simulink model "TF_TrajectoireFollowing_Segment"  (R2021b)
settings: Solver=FixedStepAuto  StartTime=0.0  StopTime=100  FixedStep=sampleTime  RelTol=1e-3  EnableMultiTasking=on
values from neighbouring files (symbols this model uses):
  k_d_x = 1.5    [startSimulation.m]
  k_d_y = 1.5    [startSimulation.m]
  k_d_yaw = 1    [startSimulation.m]
  k_d_z = 0.5    [startSimulation.m]
  k_i_x = 0.01    [startSimulation.m]
  k_i_y = 0.01    [startSimulation.m]
  k_i_yaw = 0.01    [startSimulation.m]
  k_i_z = 0.01    [startSimulation.m]
  k_p_x = 1.2    [startSimulation.m]
  k_p_y = 1.5    [startSimulation.m]
  k_p_yaw = 2    [startSimulation.m]
  k_p_z = 2    [startSimulation.m]
  saturation_psi = 2    [startSimulation.m]
  saturation_x = 2    [startSimulation.m]
  saturation_y = 2    [startSimulation.m]
  saturation_z = 2    [startSimulation.m]
libraries: simulink x28, aerolibanimutils x1
settings Model: Creator=exbot  LastModifiedBy=Lenovo
settings SolverCC: AlgebraicLoopSolver=TrustRegion
settings DataIOCC: LimitDataPoints=on  ReturnWorkspaceOutputs=off
settings OptimizationCC: LifeSpan=inf  MaxStackSize=64  EfficientTunableParamExpr=on
settings DebuggingCC: ParameterTunabilityLossMsg=error  AllowSymbolicDim=off  SFUnexpectedBacktrackingDiag=warning  SFNoUnconditionalDefaultTransitionDiag=warning  SFExecutionAtInitializationDiag=none  SFMachineParentedDataDiag=warning  ArithmeticOperatorsInVariantConditions=warning
settings HardwareCC: ProdBitPerPointer=32  ProdBitPerSizeT=32  ProdBitPerPtrDiffT=32  ProdLargestAtomicFloat=None  ProdIntDivRoundTo=Undefined  ProdEndianess=Unspecified  ProdWordSize=32  ProdHWDeviceType=Generic->Unspecified (assume 32-bit Generic)
settings ModelReferenceCC: PropagateSignalLabelsOutOfModel=off
settings SFSimCC: SimUseLocalCustomCode=off  MATLABDynamicMemAlloc=off  CustomCodeUndefinedFunction=UseInterfaceOnly  SimTargetLang=C++
settings RTWCC: Description=Embedded Coder  SystemTargetFile=ert.tlc  HardwareBoard=Robot Operating System (ROS)  TLCOptions="-aInlineSetEventsForThisBaseRateFcn=TLC_FALSE -aSuppressMultiTaskScheduler=TLC_FALSE  -aRateBasedStepFcn=0"  TemplateMakefile=ert_default_tmf  RTWUseLocalCustomCode=off  Toolchain=Catkin  TargetLang=C++
settings CodeAppCC: ForceParamTrailComments=on  IgnoreCustomStorageClasses=off  OperatorAnnotations=on  SimulinkDataObjDesc=on  SFDataObjDesc=on  MATLABFcnDesc=on  InsertBlockDesc=on  StateflowObjectComments=on  MATLABSourceComments=on
settings ERTTargetCC: MultiwordLength=2048  SupportContinuousTime=on
settings ConfigComp: CovMetricSettings=dw  CovSaveCumulativeToWorkspaceVar=on  CovSaveSingleToWorkspaceVar=on  CovExternalEMLEnable=off

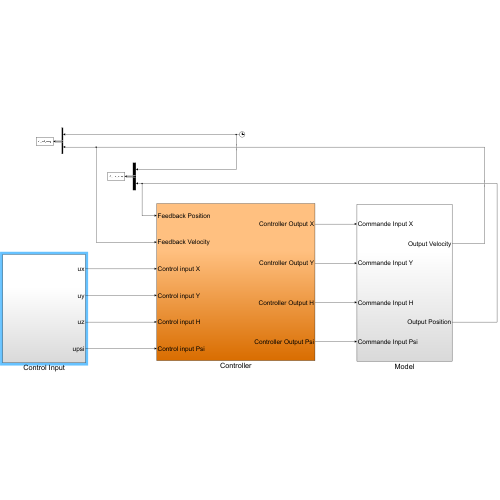
[thumbnail: Simulink's stored preview of the top-level diagram]
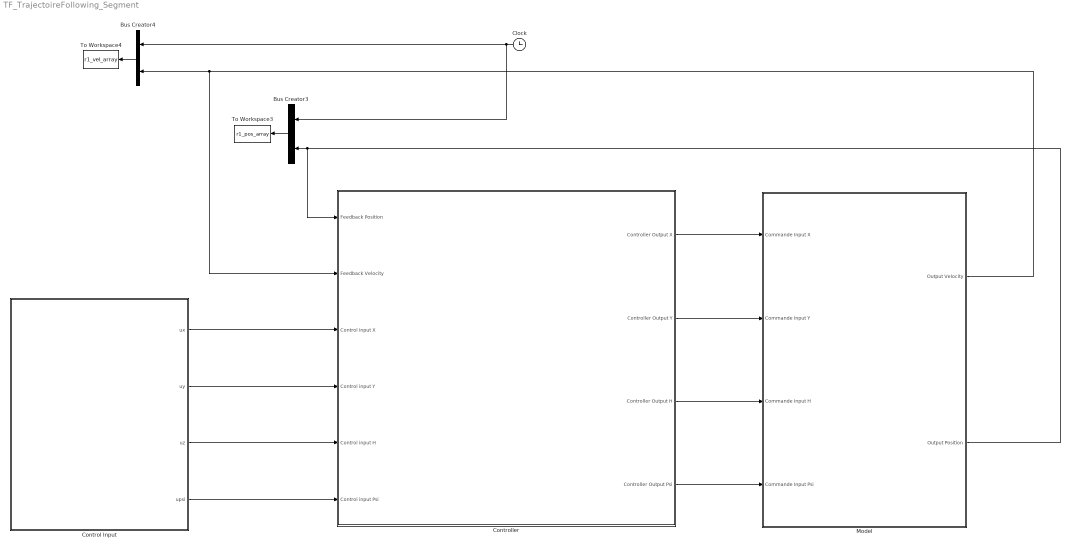
== system TF_TrajectoireFollowing_Segment ==
  Bus Creator3 : BusCreator  Inputs=2
  Bus Creator4 : BusCreator  Inputs=2
  Clock : Clock
  Control Input : Subsystem
  Controller : Subsystem
  Model : Subsystem
  To Workspace3 : ToWorkspace  VariableName=r1_pos_array  SampleTime=-1
  To Workspace4 : ToWorkspace  VariableName=r1_vel_array  SampleTime=-1
  wires:
  Clock/1 -> Bus Creator4/1, Bus Creator3/1
  Bus Creator3/1 -> To Workspace3/1
  Bus Creator4/1 -> To Workspace4/1
  Controller/1(Controller Output X) -> Model/1(Commande Input X)
  Controller/2(Controller Output Y) -> Model/2(Commande Input Y)
  Controller/3(Controller Output H) -> Model/3(Commande Input H)
  Controller/4(Controller Output Psi) -> Model/4(Commande Input Psi)
  Control Input/1(ux) -> Controller/3(Control input X)
  Control Input/2(uy) -> Controller/4(Control input Y)
  Control Input/3(uz) -> Controller/5(Control input H)
  Control Input/4(upsi) -> Controller/6(Control input Psi)
  Model/2(Output Position) -> Controller/1(Feedback Position), Bus Creator3/2
  Model/1(Output Velocity) -> Controller/2(Feedback Velocity), Bus Creator4/2

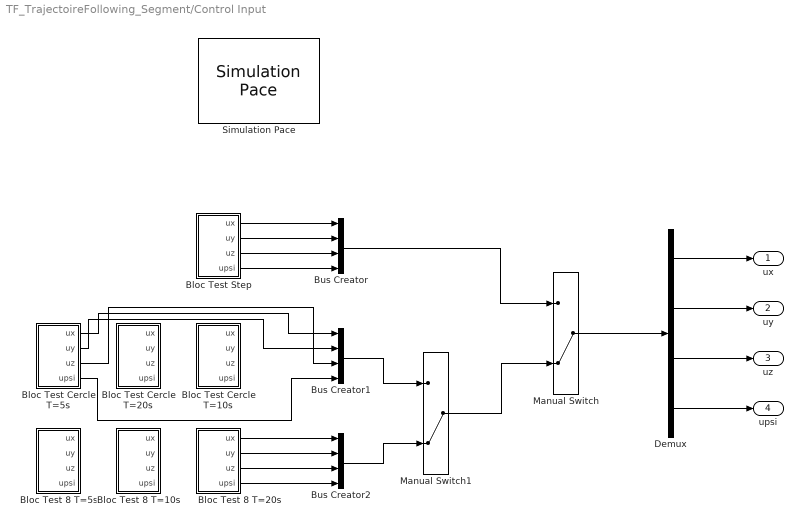
== system TF_TrajectoireFollowing_Segment/Control Input ==
  Bloc Test 8 T=10s : Subsystem
  Bloc Test 8 T=20s : Subsystem
  Bloc Test 8 T=5s : Subsystem
  Bloc Test Cercle T=10s : Subsystem
  Bloc Test Cercle T=20s : Subsystem
  Bloc Test Cercle T=5s : Subsystem
  Bloc Test Step : Subsystem
  Bus Creator : BusCreator  Inputs=4
  Bus Creator1 : BusCreator  Inputs=4
  Bus Creator2 : BusCreator  Inputs=4
  Demux : Demux
  Manual Switch : ManualSwitch  CurrentSetting=0
  Manual Switch1 : ManualSwitch  CurrentSetting=0
  Simulation Pace : aerolibanimutils/Simulation Pace  SimulationPace=100  SleepMode=MATLAB Thread  OutputPaceError=off  SampleTime=-1
  ux : Outport  VectorParamsAs1DForOutWhenUnconnected=off
  uy : Outport  Port=2  VectorParamsAs1DForOutWhenUnconnected=off
  uz : Outport  Port=3  VectorParamsAs1DForOutWhenUnconnected=off
  upsi : Outport  Port=4  VectorParamsAs1DForOutWhenUnconnected=off
  wires:
  Demux/2 -> uy/1
  Demux/1 -> ux/1
  Bloc Test Step/2(uy) -> Bus Creator/2
  Demux/3 -> uz/1
  Demux/4 -> upsi/1
  Bloc Test Step/4(upsi) -> Bus Creator/4
  Bloc Test Step/3(uz) -> Bus Creator/3
  Bloc Test Step/1(ux) -> Bus Creator/1
  Bus Creator/1 -> Manual Switch/1
  Bus Creator1/1 -> Manual Switch1/1
  Bloc Test 8 T=20s/1(ux) -> Bus Creator2/1
  Bloc Test 8 T=20s/2(uy) -> Bus Creator2/2
  Bloc Test 8 T=20s/3(uz) -> Bus Creator2/3
  Bloc Test 8 T=20s/4(upsi) -> Bus Creator2/4
  Bus Creator2/1 -> Manual Switch1/2
  Manual Switch/1 -> Demux/1
  Manual Switch1/1 -> Manual Switch/2
  Bloc Test Cercle T=5s/1(ux) -> Bus Creator1/1
  Bloc Test Cercle T=5s/2(uy) -> Bus Creator1/2
  Bloc Test Cercle T=5s/3(uz) -> Bus Creator1/3
  Bloc Test Cercle T=5s/4(upsi) -> Bus Creator1/4

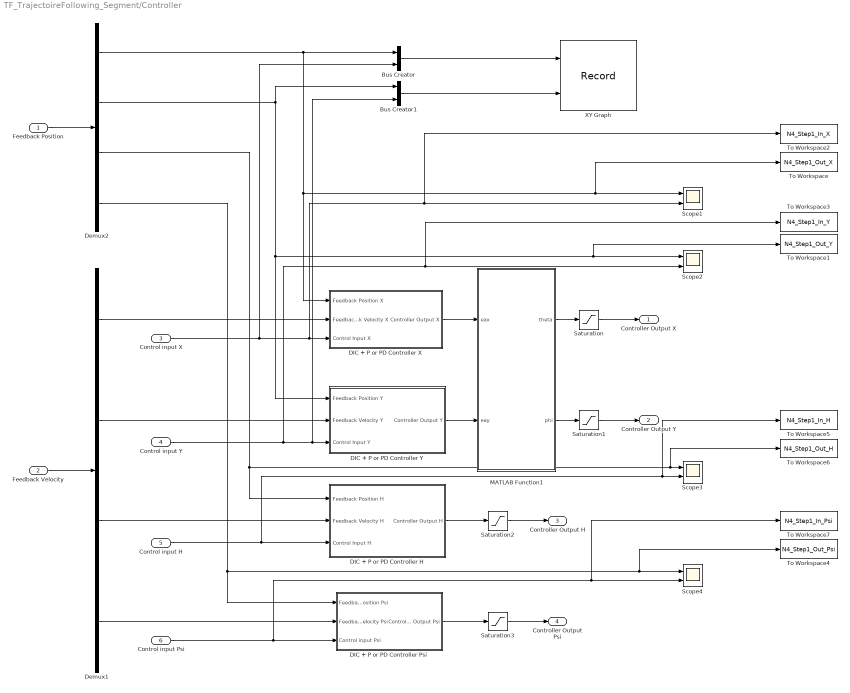
== system TF_TrajectoireFollowing_Segment/Controller ==
  Feedback Position : Inport
  Feedback Velocity : Inport  Port=2
  Control input X : Inport  Port=3
  Control input Y : Inport  Port=4
  Control input H : Inport  Port=5
  Control input Psi : Inport  Port=6
  Bus Creator : BusCreator  Inputs=2
  Bus Creator1 : BusCreator  Inputs=2
  DIC + P or PD Controller H : Subsystem
  DIC + P or PD Controller Psi : Subsystem
  DIC + P or PD Controller X : Subsystem
  DIC + P or PD Controller Y : Subsystem
  Demux1 : Demux
  Demux2 : Demux
  MATLAB Function1 : MATLAB Function  TreatAsAtomicUnit=on
  Saturation : Saturate  UpperLimit=saturation_x  LowerLimit=-saturation_x
  Saturation1 : Saturate  UpperLimit=saturation_y  LowerLimit=-saturation_y
  Saturation2 : Saturate  UpperLimit=saturation_z  LowerLimit=-saturation_z
  Saturation3 : Saturate  UpperLimit=saturation_psi  LowerLimit=-saturation_psi
  Scope{1..4} (4 alike) : Scope  NumInputPorts=2
  To Workspace : ToWorkspace  VariableName=N4_Step1_Out_X  SampleTime=-1
  To Workspace1 : ToWorkspace  VariableName=N4_Step1_Out_Y  SampleTime=-1
  To Workspace2 : ToWorkspace  VariableName=N4_Step1_In_X  SampleTime=-1
  To Workspace3 : ToWorkspace  VariableName=N4_Step1_In_Y  SampleTime=-1
  To Workspace4 : ToWorkspace  VariableName=N4_Step1_Out_Psi  SampleTime=-1
  To Workspace5 : ToWorkspace  VariableName=N4_Step1_In_H  SampleTime=-1
  To Workspace6 : ToWorkspace  VariableName=N4_Step1_Out_H  SampleTime=-1
  To Workspace7 : ToWorkspace  VariableName=N4_Step1_In_Psi  SampleTime=-1
  XY Graph : Record  FileSettingsInternal="{\"entries\":[{\"content\":{\"excelSettings\":{\"content\":{},\"type\":\"Streamout.ExcelSettings\"}},\"type\":\"Streamout.FileSettingStorage\",\"uuid\":\"f9d9ff59-c186-4da6-ac82-cd6f43ef9ca9\"}],\"packageUris\":[\"http://schema.mathworks.com/mf0/streamout_blocks/R2020a\"],\"version\":\"1.0\"}"  Layout=[1 1]  SignalsInternal="{\"entries\":[{\"content\":{\"signals\":[{\"content\":{\"blockPath\":[\"TF_TrajectoireFollowing_Segment/Controller/XY Graph\"],\"channel\":[],\"dimensions\":[1],\"domain\":\"TF_TrajectoireFollowing_Segment/Controller/XY Graph\",\"hasChildren\":true,\"lineColor\":\"#edb120\",\"plots\":[],\"port\":1,\"sid\":[\"\"],\"signalID\":78209,\"signalName\":\"Bus\\nCreator\"},\"type\":\"RecordBlkView.Signal\",\"uuid\":\"21270216-b444-45f3-8b99-29d8dc3cd5b5\"},{\"content\":{\"blockPath\":[\"TF_TrajectoireFollowing_Segment/Controller/XY Graph\"],\"channel\":[],\"dimensions\":[1],\"domain\":\"TF_TrajectoireFollowing_Segment/Controller/XY Graph\",\"leafPath\":\"Bus\\nCreator.signal1\",\"lineColor\":\"#7e2f8e\",\"parentID\":78209,\"plots\":[1],\"port\":1,\"sid\":[\"\"],\"signalID\":78215,\"signalName\":\"Bus\\nCreator.signal1\"},\"type\":\"RecordBlkView.Signal\",\"uuid\":\"6cce98a0-8777-48da-be87-494cf00595bd\"},{\"content\":{\"blockPath\":[\"TF_TrajectoireFollowing_Segment/Controller/XY Graph\"],\"channel\":[],\"dimensions\":[1],\"domain\":\"TF_TrajectoireFollowing_Segment/Controller/XY Graph\",\"leafPath\":\"Bus\\nCreator.signal2\",\"lineColor\":\"#77ac30\",\"parentID\":78209,\"plots\":[1],\"port\":1,\"sid\":[\"\"],\"signalID\":78219,\"signalName\":\"Bus\\nCreator.signal2\"},\"type\":\"RecordBlkView.Signal\",\"uuid\":\"a09ab3a8-564c-4e59-92a6-d23e7a755438\"},{\"content\":{\"blockPath\":[\"TF_TrajectoireFollowing_Segment/Controller/XY Graph\"],\"channel\":[],\"dimensions\":[1],\"domain\":\"TF_TrajectoireFollowing_Segment/Controller/XY Graph\",\"hasChildren\":true,\"lineColor\":\"#4dbeee\",\"plots\":[],\"port\":2,\"sid\":[\"\"],\"signalID\":78221,\"signalName\":\"Bus\\nCreator1\"},\"type\":\"RecordBlkView.Signal\",\"uuid\":\"b7c053ba-11ba-4e0d-9dfe-d3acde691a32\"},{\"content\":{\"blockPath\":[\"TF_TrajectoireFollowing_Segment/Controller/XY Graph\"],\"channel\":[],\"dimensions\":[1],\"domain\":\"TF_TrajectoireFollowing_Segment/Controller/XY Graph\",\"leafPath\":\"Bus\\nCreator1.signal1\",\"lineColor\":\"#a2142f\",\"parentID\":78221,\"plots\":[1],\"port\":2,\"sid\":[\"\"],\"signalID\":78227,\"signalName\":\"Bus\\nCreator1.signal1\"},\"type\":\"RecordBlkView.Signal\",\"uuid\":\"2c3fea16-f04b-45a5-a166-53e0f9a333ed\"},{\"content\":{\"blockPath\":[\"TF_TrajectoireFollowing_Segment/Controller/XY Graph\"],\"channel\":[],\"dimensions\":[1],\"domain\":\"TF_TrajectoireFollowing_Segment/Controller/XY Graph\",\"leafPath\":\"Bus\\nCreator1.signal2\",\"lineColor\":\"#139fff\",\"parentID\":78221,\"plots\":[1],\"port\":2,\"sid\":[\"\"],\"signalID\":78231,\"signalName\":\"Bus\\nCreator1.signal2\"},\"type\":\"RecordBlkView.Signal\",\"uuid\":\"06f39e5e-9c04-4ec6-a5af-5279b5cf5902\"}]},\"type\":\"RecordBlkView.InputSignals\",\"uuid\":\"564df12a-b158-43cd-be27-f4191bf5db25\"}],\"packageUris\":[\"http://schema.mathworks.com/mf0/streamout_blocks/R2020a\"],\"version\":\"1.0\"}"  VisualizationBindings="{\"xyplotplugin\":{\"info\":[{\"series\":[{\"bindingParametersList\":[{\"parameter\":\"X-Axis\",\"signalID\":78215,\"signalName\":\"Bus\\nCreator.signal1\"},{\"parameter\":\"Y-Axis\",\"signalID\":78227,\"signalName\":\"Bus\\nCreator1.signal1\"}],\"seriesID\":601},{\"bindingParametersList\":[{\"parameter\":\"X-Axis\",\"signalID\":78219,\"signalName\":\"Bus\\nCreator.signal2\"},{\"parameter\":\"Y-Axis\",\"signalID\":78231,\"signalName\":\"Bus\\nCreator1.signal2\"}],\"seriesID\":286}],\"subplotID\":1}]}}"  CompatibilityTag=XY
  Controller Output X : Outport  VectorParamsAs1DForOutWhenUnconnected=off
  Controller Output Y : Outport  Port=2  VectorParamsAs1DForOutWhenUnconnected=off
  Controller Output H : Outport  Port=3  VectorParamsAs1DForOutWhenUnconnected=off
  Controller Output Psi : Outport  Port=4  VectorParamsAs1DForOutWhenUnconnected=off
  wires:
  Feedback Position/1 -> Demux2/1
  Feedback Velocity/1 -> Demux1/1
  Demux1/2 -> DIC + P or PD Controller Y/2(Feedback Velocity Y)
  Demux2/3 -> Scope3/1, To Workspace6/1, DIC + P or PD Controller H/1(Feedback Position H)
  Demux1/1 -> DIC + P or PD Controller X/2(Feedback Velocity X)
  Demux1/3 -> DIC + P or PD Controller H/2(Feedback Velocity H)
  Control input X/1 -> Bus Creator/2, DIC + P or PD Controller X/3(Control Input X), To Workspace2/1, Scope1/2
  Control input H/1 -> Scope3/2, To Workspace5/1, DIC + P or PD Controller H/3(Control Input H)
  Saturation/1 -> Controller Output X/1
  Saturation1/1 -> Controller Output Y/1
  Saturation2/1 -> Controller Output H/1
  Saturation3/1 -> Controller Output Psi/1
  Control input Y/1 -> Bus Creator1/2, DIC + P or PD Controller Y/3(Control Input Y), Scope2/2, To Workspace3/1
  DIC + P or PD Controller H/1(Controller Output H) -> Saturation2/1
  DIC + P or PD Controller Psi/1(Controller Output Psi) -> Saturation3/1
  Demux2/1 -> Bus Creator/1, DIC + P or PD Controller X/1(Feedback Position X), To Workspace/1, Scope1/1
  Demux2/2 -> Bus Creator1/1, Scope2/1, To Workspace1/1, DIC + P or PD Controller Y/1(Feedback Position Y)
  Demux2/4 -> Scope4/1, To Workspace4/1, DIC + P or PD Controller Psi/1(Feedback Position Psi)
  Demux1/4 -> DIC + P or PD Controller Psi/2(Feedback Velocity Psi)
  Control input Psi/1 -> Scope4/2, To Workspace7/1, DIC + P or PD Controller Psi/3(Control input Psi)
  DIC + P or PD Controller Y/1(Controller Output Y) -> MATLAB Function1/2(eay)
  MATLAB Function1/2(phi) -> Saturation1/1
  DIC + P or PD Controller X/1(Controller Output X) -> MATLAB Function1/1(eax)
  MATLAB Function1/1(theta) -> Saturation/1
  Bus Creator/1 -> XY Graph/1
  Bus Creator1/1 -> XY Graph/2

== system TF_TrajectoireFollowing_Segment/Model ==
  Commande Input X : Inport
  Commande Input Y : Inport  Port=2
  Commande Input H : Inport  Port=3
  Commande Input Psi : Inport  Port=4
  Step2_Model : Subsystem
  Output Velocity : Outport  VectorParamsAs1DForOutWhenUnconnected=off
  Output Position : Outport  Port=2  VectorParamsAs1DForOutWhenUnconnected=off
  wires:
  Commande Input Y/1 -> Step2_Model/2(In2)
  Commande Input Psi/1 -> Step2_Model/4(In4)
  Commande Input H/1 -> Step2_Model/3(In3)
  Step2_Model/1(Position) -> Output Position/1
  Commande Input X/1 -> Step2_Model/1(In1)
  Step2_Model/2(Velocity) -> Output Velocity/1

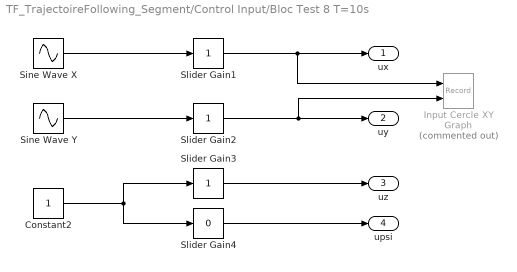
== system TF_TrajectoireFollowing_Segment/Control Input/Bloc Test 8 T=10s ==
  Constant2 : Constant
  Input Cercle XY Graph : Record  Commented=on  FileSettingsInternal="{\"entries\":[{\"content\":{\"excelSettings\":{\"content\":{},\"type\":\"Streamout.ExcelSettings\"}},\"type\":\"Streamout.FileSettingStorage\",\"uuid\":\"c4616228-9442-4d5d-9d21-8391b6b13516\"}],\"packageUris\":[\"http://schema.mathworks.com/mf0/streamout_blocks/R2020a\"],\"version\":\"1.0\"}"  Layout=[1 1]  SignalsInternal="{\"entries\":[{\"content\":{\"signals\":[{\"content\":{\"blockPath\":[\"TF_TrajectoireFollowing_Segment/Control Input/Bloc Test  8 T=10s/Input Cercle XY Graph\"],\"channel\":[],\"dimensions\":[1],\"domain\":\"TF_TrajectoireFollowing_Segment/Control Input/Bloc Test  8 T=10s/Input Cercle XY Graph\",\"lineColor\":\"#a2142f\",\"plots\":[1],\"port\":1,\"sid\":[],\"signalID\":76590,\"signalName\":\"XY Graph:1\"},\"type\":\"RecordBlkView.Signal\",\"uuid\":\"03b61a93-6194-4ac0-9fbd-1289f46fdd7e\"},{\"content\":{\"blockPath\":[\"TF_TrajectoireFollowing_Segment/Control Input/Bloc Test  8 T=10s/Input Cercle XY Graph\"],\"channel\":[],\"dimensions\":[1],\"domain\":\"TF_TrajectoireFollowing_Segment/Control Input/Bloc Test  8 T=10s/Input Cercle XY Graph\",\"lineColor\":\"#139fff\",\"plots\":[1],\"port\":2,\"sid\":[],\"signalID\":76593,\"signalName\":\"XY Graph:2\"},\"type\":\"RecordBlkView.Signal\",\"uuid\":\"b79dca94-8e28-4916-9068-c9f63d9fd3b6\"}]},\"type\":\"RecordBlkView.InputSignals\",\"uuid\":\"2ac0226d-2652-490d-8182-08a6f8622010\"}],\"packageUris\":[\"http://schema.mathworks.com/mf0/streamout_blocks/R2020a\"],\"version\":\"1.0\"}"  VisualizationBindings="{\"xyplotplugin\":{\"info\":[{\"series\":[{\"bindingParametersList\":[{\"parameter\":\"X-Axis\",\"signalID\":76590,\"signalName\":\"XY Graph:1\"},{\"parameter\":\"Y-Axis\",\"signalID\":76593,\"signalName\":\"XY Graph:2\"}],\"seriesID\":29661}],\"subplotID\":1}]}}"  CompatibilityTag=XY  st=-1
  Sine Wave X : Sin  Frequency=0.65  SampleTime=0
  Sine Wave Y : Sin  Frequency=1.3  SampleTime=0
  Slider Gain1 : simulink/Math Operations/Slider Gain  gain=1  low=-10  high=10
  Slider Gain2 : simulink/Math Operations/Slider Gain  gain=1  low=-10  high=10
  Slider Gain3 : simulink/Math Operations/Slider Gain  gain=1  low=-3  high=3
  Slider Gain4 : simulink/Math Operations/Slider Gain  gain=0  low=-2  high=2
  ux : Outport  VectorParamsAs1DForOutWhenUnconnected=off
  uy : Outport  Port=2  VectorParamsAs1DForOutWhenUnconnected=off
  uz : Outport  Port=3  VectorParamsAs1DForOutWhenUnconnected=off
  upsi : Outport  Port=4  VectorParamsAs1DForOutWhenUnconnected=off
  wires:
  Slider Gain2/1 -> Input Cercle XY Graph/2, uy/1
  Slider Gain3/1 -> uz/1
  Slider Gain4/1 -> upsi/1
  Slider Gain1/1 -> Input Cercle XY Graph/1, ux/1
  Constant2/1 -> Slider Gain4/1, Slider Gain3/1
  Sine Wave Y/1 -> Slider Gain2/1
  Sine Wave X/1 -> Slider Gain1/1

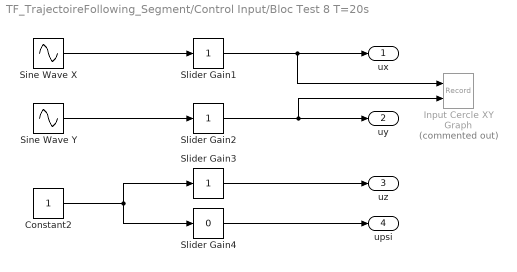
== system TF_TrajectoireFollowing_Segment/Control Input/Bloc Test 8 T=20s ==
  Constant2 : Constant
  Input Cercle XY Graph : Record  Commented=on  FileSettingsInternal="{\"entries\":[{\"content\":{\"excelSettings\":{\"content\":{},\"type\":\"Streamout.ExcelSettings\"}},\"type\":\"Streamout.FileSettingStorage\",\"uuid\":\"76c6f109-e4fe-4fb6-9c69-41c085f80ba6\"}],\"packageUris\":[\"http://schema.mathworks.com/mf0/streamout_blocks/R2020a\"],\"version\":\"1.0\"}"  Layout=[1 1]  SignalsInternal="{\"entries\":[{\"content\":{\"signals\":[{\"content\":{\"blockPath\":[\"TF_TrajectoireFollowing_Segment/Control Input/Bloc Test  8 T=20s/Input Cercle XY Graph\"],\"channel\":[],\"dimensions\":[1],\"domain\":\"TF_TrajectoireFollowing_Segment/Control Input/Bloc Test  8 T=20s/Input Cercle XY Graph\",\"lineColor\":\"#a2142f\",\"plots\":[1],\"port\":1,\"sid\":[],\"signalID\":76598,\"signalName\":\"XY Graph:1\"},\"type\":\"RecordBlkView.Signal\",\"uuid\":\"60365ea0-74d2-45aa-9d2c-46ed6597165b\"},{\"content\":{\"blockPath\":[\"TF_TrajectoireFollowing_Segment/Control Input/Bloc Test  8 T=20s/Input Cercle XY Graph\"],\"channel\":[],\"dimensions\":[1],\"domain\":\"TF_TrajectoireFollowing_Segment/Control Input/Bloc Test  8 T=20s/Input Cercle XY Graph\",\"lineColor\":\"#139fff\",\"plots\":[1],\"port\":2,\"sid\":[],\"signalID\":76601,\"signalName\":\"XY Graph:2\"},\"type\":\"RecordBlkView.Signal\",\"uuid\":\"cb74046c-3072-4053-b456-684216556246\"}]},\"type\":\"RecordBlkView.InputSignals\",\"uuid\":\"127d045c-c428-4c15-adbe-4d09a555c23a\"}],\"packageUris\":[\"http://schema.mathworks.com/mf0/streamout_blocks/R2020a\"],\"version\":\"1.0\"}"  VisualizationBindings="{\"xyplotplugin\":{\"info\":[{\"series\":[{\"bindingParametersList\":[{\"parameter\":\"X-Axis\",\"signalID\":76598,\"signalName\":\"XY Graph:1\"},{\"parameter\":\"Y-Axis\",\"signalID\":76601,\"signalName\":\"XY Graph:2\"}],\"seriesID\":37163}],\"subplotID\":1}]}}"  CompatibilityTag=XY  st=-1
  Sine Wave X : Sin  Frequency=0.35  SampleTime=0
  Sine Wave Y : Sin  Frequency=0.7  SampleTime=0
  Slider Gain1 : simulink/Math Operations/Slider Gain  gain=1  low=-10  high=10
  Slider Gain2 : simulink/Math Operations/Slider Gain  gain=1  low=-10  high=10
  Slider Gain3 : simulink/Math Operations/Slider Gain  gain=1  low=-3  high=3
  Slider Gain4 : simulink/Math Operations/Slider Gain  gain=0  low=-2  high=2
  ux : Outport  VectorParamsAs1DForOutWhenUnconnected=off
  uy : Outport  Port=2  VectorParamsAs1DForOutWhenUnconnected=off
  uz : Outport  Port=3  VectorParamsAs1DForOutWhenUnconnected=off
  upsi : Outport  Port=4  VectorParamsAs1DForOutWhenUnconnected=off
  wires:
  Slider Gain2/1 -> Input Cercle XY Graph/2, uy/1
  Slider Gain3/1 -> uz/1
  Slider Gain4/1 -> upsi/1
  Slider Gain1/1 -> Input Cercle XY Graph/1, ux/1
  Constant2/1 -> Slider Gain4/1, Slider Gain3/1
  Sine Wave Y/1 -> Slider Gain2/1
  Sine Wave X/1 -> Slider Gain1/1

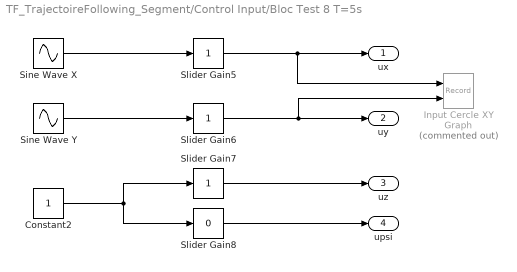
== system TF_TrajectoireFollowing_Segment/Control Input/Bloc Test 8 T=5s ==
  Constant2 : Constant
  Input Cercle XY Graph : Record  Commented=on  FileSettingsInternal="{\"entries\":[{\"content\":{\"excelSettings\":{\"content\":{},\"type\":\"Streamout.ExcelSettings\"}},\"type\":\"Streamout.FileSettingStorage\",\"uuid\":\"2a20060e-f733-4b72-afce-4417f7fccb0b\"}],\"packageUris\":[\"http://schema.mathworks.com/mf0/streamout_blocks/R2020a\"],\"version\":\"1.0\"}"  Layout=[1 1]  SignalsInternal="{\"entries\":[{\"content\":{\"signals\":[{\"content\":{\"blockPath\":[\"TF_TrajectoireFollowing_Segment/Control Input/Bloc Test  8 T=5s/Input Cercle XY Graph\"],\"channel\":[],\"dimensions\":[1],\"domain\":\"TF_TrajectoireFollowing_Segment/Control Input/Bloc Test  8 T=5s/Input Cercle XY Graph\",\"lineColor\":\"#a2142f\",\"plots\":[1],\"port\":1,\"sid\":[],\"signalID\":76606,\"signalName\":\"XY Graph:1\"},\"type\":\"RecordBlkView.Signal\",\"uuid\":\"4df2b160-309a-49c7-ba2d-556b4d832dbd\"},{\"content\":{\"blockPath\":[\"TF_TrajectoireFollowing_Segment/Control Input/Bloc Test  8 T=5s/Input Cercle XY Graph\"],\"channel\":[],\"dimensions\":[1],\"domain\":\"TF_TrajectoireFollowing_Segment/Control Input/Bloc Test  8 T=5s/Input Cercle XY Graph\",\"lineColor\":\"#139fff\",\"plots\":[1],\"port\":2,\"sid\":[],\"signalID\":76609,\"signalName\":\"XY Graph:2\"},\"type\":\"RecordBlkView.Signal\",\"uuid\":\"a6b6f2f5-6c09-4ebc-81f2-17c8bcf68424\"}]},\"type\":\"RecordBlkView.InputSignals\",\"uuid\":\"fbf89db6-4640-4c21-968e-d2b3354540fd\"}],\"packageUris\":[\"http://schema.mathworks.com/mf0/streamout_blocks/R2020a\"],\"version\":\"1.0\"}"  VisualizationBindings="{\"xyplotplugin\":{\"info\":[{\"series\":[{\"bindingParametersList\":[{\"parameter\":\"X-Axis\",\"signalID\":76606,\"signalName\":\"XY Graph:1\"},{\"parameter\":\"Y-Axis\",\"signalID\":76609,\"signalName\":\"XY Graph:2\"}],\"seriesID\":37458}],\"subplotID\":1}]}}"  CompatibilityTag=XY  st=-1
  Sine Wave X : Sin  SampleTime=0
  Sine Wave Y : Sin  Frequency=2  SampleTime=0
  Slider Gain5 : simulink/Math Operations/Slider Gain  gain=1  low=-10  high=10
  Slider Gain6 : simulink/Math Operations/Slider Gain  gain=1  low=-10  high=10
  Slider Gain7 : simulink/Math Operations/Slider Gain  gain=1  low=-3  high=3
  Slider Gain8 : simulink/Math Operations/Slider Gain  gain=0  low=-2  high=2
  ux : Outport  VectorParamsAs1DForOutWhenUnconnected=off
  uy : Outport  Port=2  VectorParamsAs1DForOutWhenUnconnected=off
  uz : Outport  Port=3  VectorParamsAs1DForOutWhenUnconnected=off
  upsi : Outport  Port=4  VectorParamsAs1DForOutWhenUnconnected=off
  wires:
  Slider Gain6/1 -> Input Cercle XY Graph/2, uy/1
  Slider Gain7/1 -> uz/1
  Slider Gain8/1 -> upsi/1
  Slider Gain5/1 -> Input Cercle XY Graph/1, ux/1
  Constant2/1 -> Slider Gain8/1, Slider Gain7/1
  Sine Wave Y/1 -> Slider Gain6/1
  Sine Wave X/1 -> Slider Gain5/1

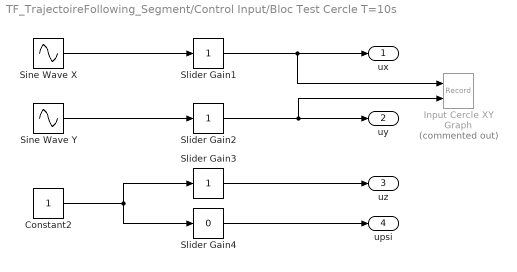
== system TF_TrajectoireFollowing_Segment/Control Input/Bloc Test Cercle T=10s ==
  Constant2 : Constant
  Input Cercle XY Graph : Record  Commented=on  FileSettingsInternal="{\"entries\":[{\"content\":{\"excelSettings\":{\"content\":{},\"type\":\"Streamout.ExcelSettings\"}},\"type\":\"Streamout.FileSettingStorage\",\"uuid\":\"2ccd6f09-7f4b-44e5-a9c2-25654386dc05\"}],\"packageUris\":[\"http://schema.mathworks.com/mf0/streamout_blocks/R2020a\"],\"version\":\"1.0\"}"  Layout=[1 1]  SignalsInternal="{\"entries\":[{\"content\":{\"signals\":[{\"content\":{\"blockPath\":[\"TF_TrajectoireFollowing_Segment/Control Input/Bloc Test  Cercle T=10s/Input Cercle XY Graph\"],\"channel\":[],\"dimensions\":[1],\"domain\":\"TF_TrajectoireFollowing_Segment/Control Input/Bloc Test  Cercle T=10s/Input Cercle XY Graph\",\"lineColor\":\"#a2142f\",\"plots\":[1],\"port\":1,\"sid\":[],\"signalID\":76614,\"signalName\":\"XY Graph:1\"},\"type\":\"RecordBlkView.Signal\",\"uuid\":\"a2f0158d-fcd9-4c4f-9076-2eb0bad3ff96\"},{\"content\":{\"blockPath\":[\"TF_TrajectoireFollowing_Segment/Control Input/Bloc Test  Cercle T=10s/Input Cercle XY Graph\"],\"channel\":[],\"dimensions\":[1],\"domain\":\"TF_TrajectoireFollowing_Segment/Control Input/Bloc Test  Cercle T=10s/Input Cercle XY Graph\",\"lineColor\":\"#139fff\",\"plots\":[1],\"port\":2,\"sid\":[],\"signalID\":76617,\"signalName\":\"XY Graph:2\"},\"type\":\"RecordBlkView.Signal\",\"uuid\":\"a3d89165-7dc3-4862-9d2a-9a3121fc1798\"}]},\"type\":\"RecordBlkView.InputSignals\",\"uuid\":\"9116e90b-d238-4373-b271-860144c3e8b5\"}],\"packageUris\":[\"http://schema.mathworks.com/mf0/streamout_blocks/R2020a\"],\"version\":\"1.0\"}"  VisualizationBindings="{\"xyplotplugin\":{\"info\":[{\"series\":[{\"bindingParametersList\":[{\"parameter\":\"X-Axis\",\"signalID\":76614,\"signalName\":\"XY Graph:1\"},{\"parameter\":\"Y-Axis\",\"signalID\":76617,\"signalName\":\"XY Graph:2\"}],\"seriesID\":58776}],\"subplotID\":1}]}}"  CompatibilityTag=XY  st=-1
  Sine Wave X : Sin  Frequency=0.65  SampleTime=0
  Sine Wave Y : Sin  Frequency=0.65  Phase=pi/2  SampleTime=0
  Slider Gain1 : simulink/Math Operations/Slider Gain  gain=1  low=-10  high=10
  Slider Gain2 : simulink/Math Operations/Slider Gain  gain=1  low=-10  high=10
  Slider Gain3 : simulink/Math Operations/Slider Gain  gain=1  low=-3  high=3
  Slider Gain4 : simulink/Math Operations/Slider Gain  gain=0  low=-2  high=2
  ux : Outport  VectorParamsAs1DForOutWhenUnconnected=off
  uy : Outport  Port=2  VectorParamsAs1DForOutWhenUnconnected=off
  uz : Outport  Port=3  VectorParamsAs1DForOutWhenUnconnected=off
  upsi : Outport  Port=4  VectorParamsAs1DForOutWhenUnconnected=off
  wires:
  Slider Gain2/1 -> Input Cercle XY Graph/2, uy/1
  Slider Gain3/1 -> uz/1
  Slider Gain4/1 -> upsi/1
  Slider Gain1/1 -> Input Cercle XY Graph/1, ux/1
  Constant2/1 -> Slider Gain4/1, Slider Gain3/1
  Sine Wave Y/1 -> Slider Gain2/1
  Sine Wave X/1 -> Slider Gain1/1

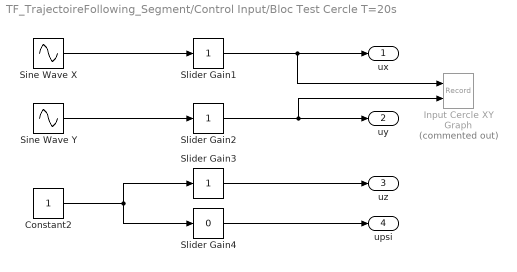
== system TF_TrajectoireFollowing_Segment/Control Input/Bloc Test Cercle T=20s ==
  Constant2 : Constant
  Input Cercle XY Graph : Record  Commented=on  FileSettingsInternal="{\"entries\":[{\"content\":{\"excelSettings\":{\"content\":{},\"type\":\"Streamout.ExcelSettings\"}},\"type\":\"Streamout.FileSettingStorage\",\"uuid\":\"f27aa7e8-62ac-4aa5-b51d-eb7641399cc6\"}],\"packageUris\":[\"http://schema.mathworks.com/mf0/streamout_blocks/R2020a\"],\"version\":\"1.0\"}"  Layout=[1 1]  SignalsInternal="{\"entries\":[{\"content\":{\"signals\":[{\"content\":{\"blockPath\":[\"TF_TrajectoireFollowing_Segment/Control Input/Bloc Test  Cercle T=20s/Input Cercle XY Graph\"],\"channel\":[],\"dimensions\":[1],\"domain\":\"TF_TrajectoireFollowing_Segment/Control Input/Bloc Test  Cercle T=20s/Input Cercle XY Graph\",\"lineColor\":\"#a2142f\",\"plots\":[1],\"port\":1,\"sid\":[],\"signalID\":76622,\"signalName\":\"XY Graph:1\"},\"type\":\"RecordBlkView.Signal\",\"uuid\":\"2086e63e-339f-4229-a288-c28a1e172dd9\"},{\"content\":{\"blockPath\":[\"TF_TrajectoireFollowing_Segment/Control Input/Bloc Test  Cercle T=20s/Input Cercle XY Graph\"],\"channel\":[],\"dimensions\":[1],\"domain\":\"TF_TrajectoireFollowing_Segment/Control Input/Bloc Test  Cercle T=20s/Input Cercle XY Graph\",\"lineColor\":\"#139fff\",\"plots\":[1],\"port\":2,\"sid\":[],\"signalID\":76625,\"signalName\":\"XY Graph:2\"},\"type\":\"RecordBlkView.Signal\",\"uuid\":\"7ec62dda-8496-467e-a243-f75a2a8c807b\"}]},\"type\":\"RecordBlkView.InputSignals\",\"uuid\":\"33839adb-f547-45c6-94eb-e0907bfb8c7b\"}],\"packageUris\":[\"http://schema.mathworks.com/mf0/streamout_blocks/R2020a\"],\"version\":\"1.0\"}"  VisualizationBindings="{\"xyplotplugin\":{\"info\":[{\"series\":[{\"bindingParametersList\":[{\"parameter\":\"X-Axis\",\"signalID\":76622,\"signalName\":\"XY Graph:1\"},{\"parameter\":\"Y-Axis\",\"signalID\":76625,\"signalName\":\"XY Graph:2\"}],\"seriesID\":62067}],\"subplotID\":1}]}}"  CompatibilityTag=XY  st=-1
  Sine Wave X : Sin  Frequency=0.35  SampleTime=0
  Sine Wave Y : Sin  Frequency=0.35  Phase=pi/2  SampleTime=0
  Slider Gain1 : simulink/Math Operations/Slider Gain  gain=1  low=-10  high=10
  Slider Gain2 : simulink/Math Operations/Slider Gain  gain=1  low=-10  high=10
  Slider Gain3 : simulink/Math Operations/Slider Gain  gain=1  low=-3  high=3
  Slider Gain4 : simulink/Math Operations/Slider Gain  gain=0  low=-2  high=2
  ux : Outport  VectorParamsAs1DForOutWhenUnconnected=off
  uy : Outport  Port=2  VectorParamsAs1DForOutWhenUnconnected=off
  uz : Outport  Port=3  VectorParamsAs1DForOutWhenUnconnected=off
  upsi : Outport  Port=4  VectorParamsAs1DForOutWhenUnconnected=off
  wires:
  Slider Gain2/1 -> Input Cercle XY Graph/2, uy/1
  Slider Gain3/1 -> uz/1
  Slider Gain4/1 -> upsi/1
  Slider Gain1/1 -> Input Cercle XY Graph/1, ux/1
  Constant2/1 -> Slider Gain4/1, Slider Gain3/1
  Sine Wave Y/1 -> Slider Gain2/1
  Sine Wave X/1 -> Slider Gain1/1

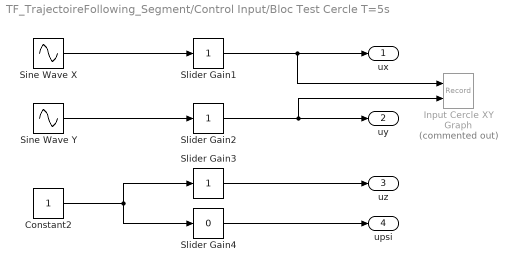
== system TF_TrajectoireFollowing_Segment/Control Input/Bloc Test Cercle T=5s ==
  Constant2 : Constant
  Input Cercle XY Graph : Record  Commented=on  FileSettingsInternal="{\"entries\":[{\"content\":{\"excelSettings\":{\"content\":{},\"type\":\"Streamout.ExcelSettings\"}},\"type\":\"Streamout.FileSettingStorage\",\"uuid\":\"c0d29a17-4a30-4159-b996-24eac29678bd\"}],\"packageUris\":[\"http://schema.mathworks.com/mf0/streamout_blocks/R2020a\"],\"version\":\"1.0\"}"  Layout=[1 1]  SignalsInternal="{\"entries\":[{\"content\":{\"signals\":[{\"content\":{\"blockPath\":[\"TF_TrajectoireFollowing_Segment/Control Input/Bloc Test  Cercle T=5s/Input Cercle XY Graph\"],\"channel\":[],\"dimensions\":[1],\"domain\":\"TF_TrajectoireFollowing_Segment/Control Input/Bloc Test  Cercle T=5s/Input Cercle XY Graph\",\"lineColor\":\"#a2142f\",\"plots\":[1],\"port\":1,\"sid\":[],\"signalID\":76630,\"signalName\":\"XY Graph:1\"},\"type\":\"RecordBlkView.Signal\",\"uuid\":\"424d9596-8aa7-474d-a03d-5a545e7a330b\"},{\"content\":{\"blockPath\":[\"TF_TrajectoireFollowing_Segment/Control Input/Bloc Test  Cercle T=5s/Input Cercle XY Graph\"],\"channel\":[],\"dimensions\":[1],\"domain\":\"TF_TrajectoireFollowing_Segment/Control Input/Bloc Test  Cercle T=5s/Input Cercle XY Graph\",\"lineColor\":\"#139fff\",\"plots\":[1],\"port\":2,\"sid\":[],\"signalID\":76633,\"signalName\":\"XY Graph:2\"},\"type\":\"RecordBlkView.Signal\",\"uuid\":\"33db0850-10b5-4170-880b-d9faeec5613f\"}]},\"type\":\"RecordBlkView.InputSignals\",\"uuid\":\"a83120cd-5245-4f79-8e4b-4a8e1e05b58d\"}],\"packageUris\":[\"http://schema.mathworks.com/mf0/streamout_blocks/R2020a\"],\"version\":\"1.0\"}"  VisualizationBindings="{\"xyplotplugin\":{\"info\":[{\"series\":[{\"bindingParametersList\":[{\"parameter\":\"X-Axis\",\"signalID\":76630,\"signalName\":\"XY Graph:1\"},{\"parameter\":\"Y-Axis\",\"signalID\":76633,\"signalName\":\"XY Graph:2\"}],\"seriesID\":15496}],\"subplotID\":1}]}}"  CompatibilityTag=XY  st=-1
  Sine Wave X : Sin  SampleTime=0
  Sine Wave Y : Sin  Phase=pi/2  SampleTime=0
  Slider Gain1 : simulink/Math Operations/Slider Gain  gain=1  low=-10  high=10
  Slider Gain2 : simulink/Math Operations/Slider Gain  gain=1  low=-10  high=10
  Slider Gain3 : simulink/Math Operations/Slider Gain  gain=1  low=-3  high=3
  Slider Gain4 : simulink/Math Operations/Slider Gain  gain=0  low=-2  high=2
  ux : Outport  VectorParamsAs1DForOutWhenUnconnected=off
  uy : Outport  Port=2  VectorParamsAs1DForOutWhenUnconnected=off
  uz : Outport  Port=3  VectorParamsAs1DForOutWhenUnconnected=off
  upsi : Outport  Port=4  VectorParamsAs1DForOutWhenUnconnected=off
  wires:
  Slider Gain2/1 -> Input Cercle XY Graph/2, uy/1
  Slider Gain3/1 -> uz/1
  Slider Gain4/1 -> upsi/1
  Slider Gain1/1 -> Input Cercle XY Graph/1, ux/1
  Constant2/1 -> Slider Gain4/1, Slider Gain3/1
  Sine Wave Y/1 -> Slider Gain2/1
  Sine Wave X/1 -> Slider Gain1/1

== system TF_TrajectoireFollowing_Segment/Control Input/Bloc Test Step ==
  Constant2 : Constant
  Input Segment XY Graph : Record  Commented=on  FileSettingsInternal="{\"entries\":[{\"content\":{\"excelSettings\":{\"content\":{},\"type\":\"Streamout.ExcelSettings\"}},\"type\":\"Streamout.FileSettingStorage\",\"uuid\":\"6933d473-09aa-4c90-8556-9d3b1625d3cb\"}],\"packageUris\":[\"http://schema.mathworks.com/mf0/streamout_blocks/R2020a\"],\"version\":\"1.0\"}"  Layout=[1 1]  SignalsInternal="{\"entries\":[{\"content\":{\"signals\":[{\"content\":{\"blockPath\":[\"TF_TrajectoireFollowing_Segment/Control Input/Bloc Test  Step/Input Segment XY Graph\"],\"channel\":[],\"dimensions\":[1],\"domain\":\"TF_TrajectoireFollowing_Segment/Control Input/Bloc Test  Step/Input Segment XY Graph\",\"lineColor\":\"#a2142f\",\"plots\":[1],\"port\":1,\"sid\":[],\"signalID\":76638,\"signalName\":\"XY Graph:1\"},\"type\":\"RecordBlkView.Signal\",\"uuid\":\"501e8f4e-48af-4e7c-a96d-4f4b1c663e78\"},{\"content\":{\"blockPath\":[\"TF_TrajectoireFollowing_Segment/Control Input/Bloc Test  Step/Input Segment XY Graph\"],\"channel\":[],\"dimensions\":[1],\"domain\":\"TF_TrajectoireFollowing_Segment/Control Input/Bloc Test  Step/Input Segment XY Graph\",\"lineColor\":\"#139fff\",\"plots\":[1],\"port\":2,\"sid\":[],\"signalID\":76641,\"signalName\":\"XY Graph:2\"},\"type\":\"RecordBlkView.Signal\",\"uuid\":\"826c3666-f92a-4d49-8303-b3d7bbd3b006\"}]},\"type\":\"RecordBlkView.InputSignals\",\"uuid\":\"0e37ff94-bf76-4b2f-83bc-0a46c8c73ef6\"}],\"packageUris\":[\"http://schema.mathworks.com/mf0/streamout_blocks/R2020a\"],\"version\":\"1.0\"}"  VisualizationBindings="{\"xyplotplugin\":{\"info\":[{\"series\":[{\"bindingParametersList\":[{\"parameter\":\"X-Axis\",\"signalID\":76638,\"signalName\":\"XY Graph:1\"},{\"parameter\":\"Y-Axis\",\"signalID\":76641,\"signalName\":\"XY Graph:2\"}],\"seriesID\":1418}],\"subplotID\":1}]}}"  CompatibilityTag=XY  st=-1
  Slider Gain1 : simulink/Math Operations/Slider Gain  gain=1  low=-10  high=10
  Slider Gain2 : simulink/Math Operations/Slider Gain  gain=1  low=-10  high=10
  Slider Gain3 : simulink/Math Operations/Slider Gain  gain=1  low=-2  high=2
  Slider Gain4 : simulink/Math Operations/Slider Gain  gain=0  low=-2  high=2
  Step X1 : Step  Time=5  SampleTime=0
  ux : Outport  VectorParamsAs1DForOutWhenUnconnected=off
  uy : Outport  Port=2  VectorParamsAs1DForOutWhenUnconnected=off
  uz : Outport  Port=3  VectorParamsAs1DForOutWhenUnconnected=off
  upsi : Outport  Port=4  VectorParamsAs1DForOutWhenUnconnected=off
  wires:
  Slider Gain1/1 -> Input Segment XY Graph/1, ux/1
  Slider Gain2/1 -> Input Segment XY Graph/2, uy/1
  Slider Gain3/1 -> uz/1
  Slider Gain4/1 -> upsi/1
  Step X1/1 -> Slider Gain3/1, Slider Gain4/1, Slider Gain2/1, Slider Gain1/1

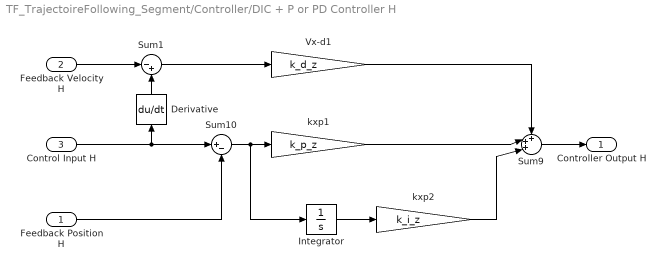
== system TF_TrajectoireFollowing_Segment/Controller/DIC + P or PD Controller H ==
  Feedback Position H : Inport
  Feedback Velocity H : Inport  Port=2
  Control Input H : Inport  Port=3
  Derivative : Derivative
  Integrator : Integrator
  Sum1 : Sum  Inputs=|-+
  Sum10 : Sum  Inputs=|+-
  Sum9 : Sum  Inputs=+++|
  Vx-d1 : Gain  Gain=k_d_z
  kxp1 : Gain  Gain=k_p_z
  kxp2 : Gain  Gain=k_i_z
  Controller Output H : Outport  VectorParamsAs1DForOutWhenUnconnected=off
  wires:
  Sum9/1 -> Controller Output H/1
  Sum10/1 -> Integrator/1, kxp1/1
  kxp1/1 -> Sum9/2
  Vx-d1/1 -> Sum9/1
  Feedback Velocity H/1 -> Sum1/1
  Sum1/1 -> Vx-d1/1
  Integrator/1 -> kxp2/1
  kxp2/1 -> Sum9/3
  Control Input H/1 -> Sum10/1, Derivative/1
  Feedback Position H/1 -> Sum10/2
  Derivative/1 -> Sum1/2

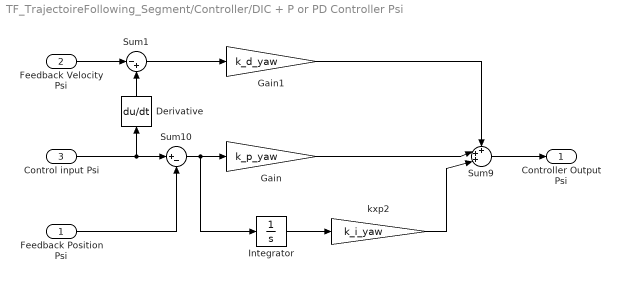
== system TF_TrajectoireFollowing_Segment/Controller/DIC + P or PD Controller Psi ==
  Feedback Position Psi : Inport
  Feedback Velocity Psi : Inport  Port=2
  Control input Psi : Inport  Port=3
  Derivative : Derivative
  Gain : Gain  Gain=k_p_yaw
  Gain1 : Gain  Gain=k_d_yaw
  Integrator : Integrator
  Sum1 : Sum  Inputs=|-+
  Sum10 : Sum  Inputs=|+-
  Sum9 : Sum  Inputs=+++|
  kxp2 : Gain  Gain=k_i_yaw
  Controller Output Psi : Outport  VectorParamsAs1DForOutWhenUnconnected=off
  wires:
  Sum9/1 -> Controller Output Psi/1
  kxp2/1 -> Sum9/3
  Control input Psi/1 -> Sum10/1, Derivative/1
  Gain1/1 -> Sum9/1
  Sum10/1 -> Gain/1, Integrator/1
  Integrator/1 -> kxp2/1
  Feedback Velocity Psi/1 -> Sum1/1
  Sum1/1 -> Gain1/1
  Gain/1 -> Sum9/2
  Derivative/1 -> Sum1/2
  Feedback Position Psi/1 -> Sum10/2

== system TF_TrajectoireFollowing_Segment/Controller/DIC + P or PD Controller X ==
  Feedback Position X : Inport
  Feedback Velocity X : Inport  Port=2
  Control Input X : Inport  Port=3
  Derivative : Derivative
  Integrator : Integrator
  Sum1 : Sum  Inputs=|-+
  Sum10 : Sum  Inputs=|+-
  Sum9 : Sum  Inputs=+++|
  Vx-d3 : Gain  Gain=k_d_x
  kxp2 : Gain  Gain=k_i_x
  kxp3 : Gain  Gain=k_p_x
  Controller Output X : Outport  VectorParamsAs1DForOutWhenUnconnected=off
  wires:
  Sum9/1 -> Controller Output X/1
  Feedback Velocity X/1 -> Sum1/1
  Feedback Position X/1 -> Sum10/2
  Sum1/1 -> Vx-d3/1
  Integrator/1 -> kxp2/1
  kxp3/1 -> Sum9/2
  Vx-d3/1 -> Sum9/1
  Sum10/1 -> kxp3/1, Integrator/1
  Derivative/1 -> Sum1/2
  kxp2/1 -> Sum9/3
  Control Input X/1 -> Sum10/1, Derivative/1

== system TF_TrajectoireFollowing_Segment/Controller/DIC + P or PD Controller Y ==
  Feedback Position Y : Inport
  Feedback Velocity Y : Inport  Port=2
  Control Input Y : Inport  Port=3
  Derivative : Derivative
  Integrator : Integrator
  Sum1 : Sum  Inputs=|-+
  Sum10 : Sum  Inputs=|+-
  Sum9 : Sum  Inputs=+++|
  Vx-d3 : Gain  Gain=k_d_y
  kxp2 : Gain  Gain=k_i_y
  kxp3 : Gain  Gain=k_p_y
  Controller Output Y : Outport  VectorParamsAs1DForOutWhenUnconnected=off
  wires:
  Feedback Position Y/1 -> Sum10/2
  Control Input Y/1 -> Sum10/1, Derivative/1
  Sum9/1 -> Controller Output Y/1
  Integrator/1 -> kxp2/1
  kxp3/1 -> Sum9/2
  Sum10/1 -> kxp3/1, Integrator/1
  kxp2/1 -> Sum9/3
  Vx-d3/1 -> Sum9/1
  Feedback Velocity Y/1 -> Sum1/1
  Sum1/1 -> Vx-d3/1
  Derivative/1 -> Sum1/2

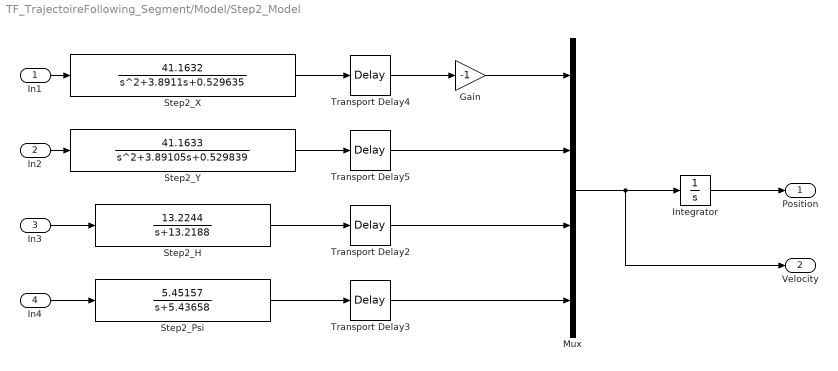
== system TF_TrajectoireFollowing_Segment/Model/Step2_Model ==
  In1 : Inport
  In2 : Inport  Port=2
  In3 : Inport  Port=3
  In4 : Inport  Port=4
  Gain : Gain  Gain=-1
  Integrator : Integrator
  Mux : Mux
  Step2_H : TransferFcn  Numerator=13.2244  Denominator=[1 13.2188]
  Step2_Psi : TransferFcn  Numerator=5.45157  Denominator=[1 5.43658]
  Step2_X : TransferFcn  Numerator=41.1632  Denominator=[1 3.8911 0.529635]
  Step2_Y : TransferFcn  Numerator=41.1633  Denominator=[1 3.89105 0.529839]
  Transport Delay2 : TransportDelay  DelayTime=0.0344
  Transport Delay3 : TransportDelay  DelayTime=0.0313
  Transport Delay4 : TransportDelay  DelayTime=0.0289
  Transport Delay5 : TransportDelay  DelayTime=0.0289
  Position : Outport  VectorParamsAs1DForOutWhenUnconnected=off
  Velocity : Outport  Port=2  VectorParamsAs1DForOutWhenUnconnected=off
  wires:
  Transport Delay2/1 -> Mux/3
  In2/1 -> Step2_Y/1
  In4/1 -> Step2_Psi/1
  Transport Delay3/1 -> Mux/4
  In1/1 -> Step2_X/1
  In3/1 -> Step2_H/1
  Step2_H/1 -> Transport Delay2/1
  Step2_Y/1 -> Transport Delay5/1
  Step2_X/1 -> Transport Delay4/1
  Step2_Psi/1 -> Transport Delay3/1
  Transport Delay4/1 -> Gain/1
  Transport Delay5/1 -> Mux/2
  Integrator/1 -> Position/1
  Mux/1 -> Velocity/1, Integrator/1
  Gain/1 -> Mux/1

== matlab function TF_TrajectoireFollowing_Segment/Controller/MATLAB Function1 ==
  data: theta output; eax input; eay input; phi output
function [theta,phi] = fcn(eax,eay)
g=9.8;

theta =-eax/g;% vx
phi =eay/g;% vy
